simulink model "PlantaInestable"  (R2017b)
settings: Solver=VariableStepAuto  StartTime=0.0  StopTime=10  RelTol=1e-3
values from neighbouring files (symbols this model uses):
  dgain_pd = polynomial_pd(2)    [Unstable_FinalProject.m]
  igain_pi = polynomial_pi(1)- pgain_pi    [Unstable_FinalProject.m]
  kc = -polynomial(2)-(2*kd)    [Unstable_FinalProject.m]
  kd = polynomial(3)    [Unstable_FinalProject.m]
  ki = polynomial(1) - kd - kc    [Unstable_FinalProject.m]
  p_gain = 12    [Unstable_FinalProject.m]
  pgain_pd = polynomial_pd(1)- dgain_pd    [Unstable_FinalProject.m]
  pgain_pi = polynomial_pi(2)    [Unstable_FinalProject.m]
  Ts = round(T,2)    [Unstable_FinalProject.m]
libraries: cstblocks x6, simulink x2
settings Model: Creator=dplascen  LastModifiedBy=dplascen

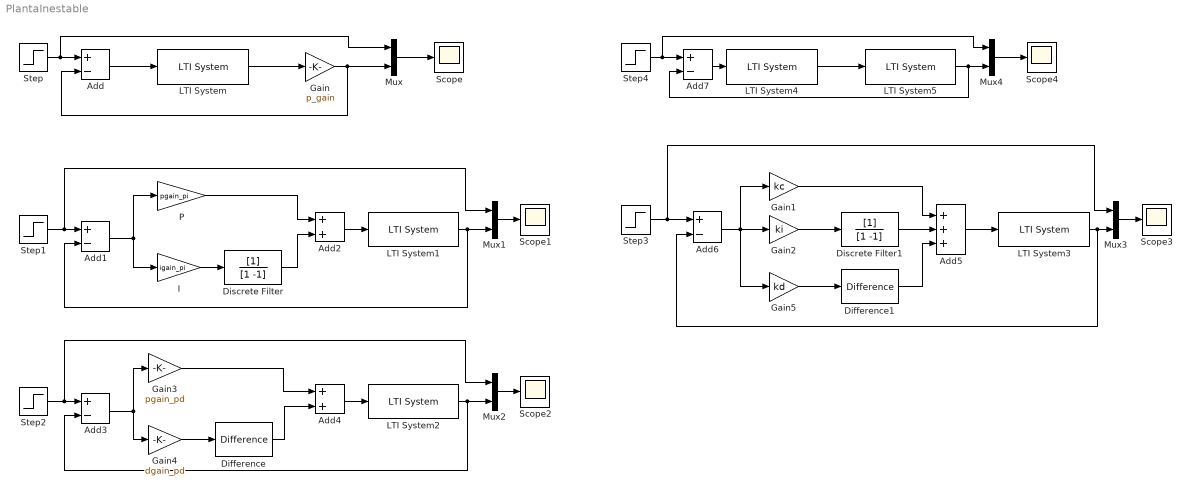
== system PlantaInestable ==
  Add{,1,3,6..7} (5 alike) : Sum  Inputs=+-
  Add2 : Sum
  Add4 : Sum
  Add5 : Sum  Inputs=+++
  Difference : simulink/Discrete/Difference  ICPrevInput=0.0  OutMin=[]  OutMax=[]  OutDataType=fixdt(1, 16)  OutScaling=2^-10  DoSatur=off
  Difference1 : simulink/Discrete/Difference  ICPrevInput=0.0  OutMin=[]  OutMax=[]  OutDataType=fixdt(1, 16)  OutScaling=2^-10  DoSatur=off
  Discrete Filter : DiscreteFilter  Denominator=[1 -1]  SampleTime=Ts
  Discrete Filter1 : DiscreteFilter  Denominator=[1 -1]  SampleTime=Ts
  Gain : Gain  Gain=p_gain
  Gain1 : Gain  Gain=kc
  Gain2 : Gain  Gain=ki
  Gain3 : Gain  Gain=pgain_pd
  Gain4 : Gain  Gain=dgain_pd
  Gain5 : Gain  Gain=kd
  I : Gain  Gain=igain_pi
  LTI System{,1..4} (5 alike) : cstblocks/LTI System  sys=Gz  IC=[]
  LTI System5 : cstblocks/LTI System  sys=C2z  IC=[]
  Mux{,1..4} (5 alike) : Mux  Inputs=2
  "P " : Gain  Gain=pgain_pi
  Scope{,1..4} (5 alike) : Scope
  Step{,1..2,4} (4 alike) : Step  SampleTime=0
  Step3 : Step  Time=0  SampleTime=0
  wires:
  LTI System/1 -> Gain/1
  Add/1 -> LTI System/1
  Step/1 -> Add/1, Mux/1
  Gain/1 -> Add/2, Mux/2
  Mux/1 -> Scope/1
  Gain3/1 -> Add4/1
  Add3/1 -> Gain3/1, Gain4/1
  Add4/1 -> LTI System2/1
  Difference/1 -> Add4/2
  Mux2/1 -> Scope2/1
  Step2/1 -> Mux2/1, Add3/1
  Gain4/1 -> Difference/1
  LTI System2/1 -> Add3/2, Mux2/2
  Add5/1 -> LTI System3/1
  Gain1/1 -> Add5/1
  Discrete Filter1/1 -> Add5/2
  Difference1/1 -> Add5/3
  Gain5/1 -> Difference1/1
  Add6/1 -> Gain1/1, Gain5/1, Gain2/1
  Mux3/1 -> Scope3/1
  Step3/1 -> Mux3/1, Add6/1
  "P "/1 -> Add2/1
  Add1/1 -> "P "/1, I/1
  Discrete Filter/1 -> Add2/2
  LTI System1/1 -> Add1/2, Mux1/2
  Add2/1 -> LTI System1/1
  Step1/1 -> Mux1/1, Add1/1
  Mux1/1 -> Scope1/1
  I/1 -> Discrete Filter/1
  Gain2/1 -> Discrete Filter1/1
  Mux4/1 -> Scope4/1
  Step4/1 -> Add7/1, Mux4/1
  Add7/1 -> LTI System4/1
  LTI System4/1 -> LTI System5/1
  LTI System5/1 -> Add7/2, Mux4/2
  LTI System3/1 -> Add6/2, Mux3/2
